simulink model "model_fallback"  (R2016a)
settings: Solver=VariableStepAuto  StartTime=0.0  StopTime=10.0  RelTol=1e-3
values from neighbouring files (symbols this model uses):
  alfa = 216.9    [init_fallback.m]
  g = 9.81    [init_fallback.m]
  L0 = 0.1255    [init_fallback.m]
  L1 = 0.05132    [init_fallback.m]
  m = 57.5    [init_fallback.m]
  R = 5.45    [init_fallback.m]
  x1zad = 0.015    [init_fallback.m]
undefined symbols (not defined in the file or in its folder): K, L
libraries: simulink x2
settings Model: Creator=Filip  LastModifiedBy=Filip

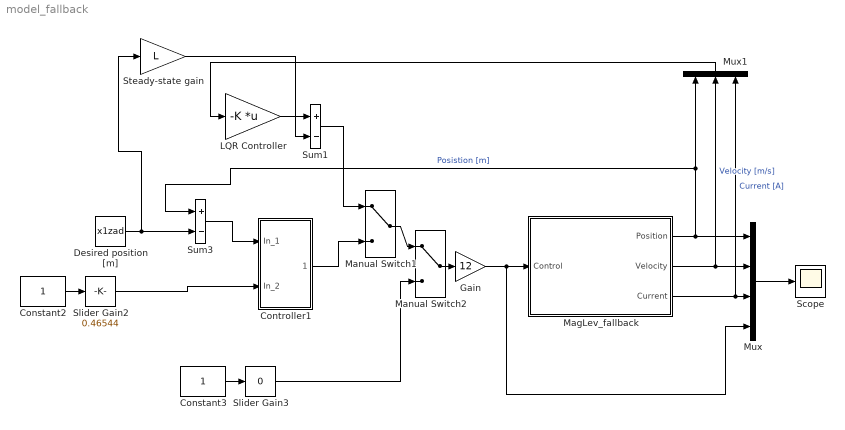
== system model_fallback ==
  Constant2 : Constant
  Constant3 : Constant
  Controller1 : Subsystem  mask(PID(2) Controller){P=40, I=3, D=0.5, T0=0.001}
      mask prompts: P "Proportional:"; I "Integral:"; D "Derivative:"; T0 "Sample Time:"
      mask help:
      | Enter Proportional(P), Integral(I), and Derivative(D) and divisor (N) terms.
      | P+I/s+Ds/(1/Ns+1)
      mask Help: This block implements a PID controller where parameters are entered for the Proportional, Integral and Derivative and divisor terms. Unmask this block to see how it works. The derivative term is implemented using an s/(s/N +1)  transfer function block. Making N large can create a "stiff" system.
      mask Display: disp('PID')
  "Desired position [m] " : Constant  Value=x1zad
  Gain : Gain  Gain=12
  LQR Controller : Gain  Gain=-K  Multiplication=Matrix(K*u)
  MagLev_fallback : Subsystem
  Manual Switch1 : ManualSwitch
  Manual Switch2 : ManualSwitch
  Mux : Mux
  Mux1 : Mux  Inputs=3
  Scope : Scope
  Slider Gain2 : simulink/Math Operations/Slider Gain  low=0  gain=0.46544  high=1
  Slider Gain3 : simulink/Math Operations/Slider Gain  low=0  gain=0  high=1
  Steady-state gain : Gain  Gain=L
  Sum1 : Sum  Inputs=+-  SaturateOnIntegerOverflow=on  InputSameDT=on  OutDataTypeStr=Inherit: Same as first input
  Sum3 : Sum  Inputs=+-  SaturateOnIntegerOverflow=on  InputSameDT=on  OutDataTypeStr=Inherit: Same as first input
  wires:
  Mux/1 -> Scope/1
  Gain/1 -> Mux/4, MagLev_fallback/1(Control)
  Manual Switch2/1 -> Gain/1
  MagLev_fallback/1(Position) -> Sum3/1, Mux1/1, Mux/1  "Posistion [m]"
  Constant2/1 -> Slider Gain2/1
  Slider Gain2/1 -> Controller1/2(In_2)
  "Desired position [m] "/1 -> Steady-state gain/1, Sum3/2
  Sum3/1 -> Controller1/1(In_1)
  Constant3/1 -> Slider Gain3/1
  Slider Gain3/1 -> Manual Switch2/2
  Manual Switch1/1 -> Manual Switch2/1
  Controller1/1(Out_1) -> Manual Switch1/2
  Mux1/1 -> LQR Controller/1
  LQR Controller/1 -> Sum1/1
  Sum1/1 -> Manual Switch1/1
  Steady-state gain/1 -> Sum1/2
  MagLev_fallback/2("Velocity ") -> Mux1/2, Mux/2  "Velocity [m/s]"
  MagLev_fallback/3(Current) -> Mux1/3, Mux/3  "Current [A]"

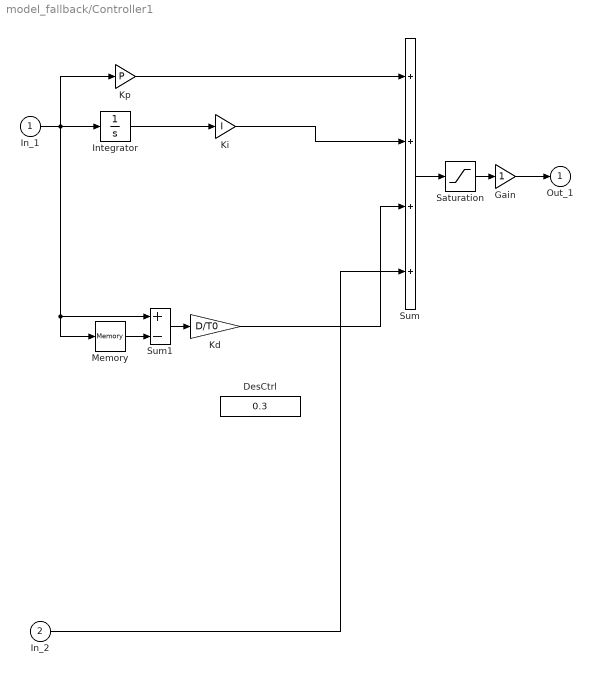
== system model_fallback/Controller1 ==
  In_1 : Inport
  In_2 : Inport  Port=2
  DesCtrl : Constant  Value=0.3
  Gain : Gain  SaturateOnIntegerOverflow=on  OutDataTypeStr=Inherit: Same as input  ParamDataTypeStr=Inherit: Same as input
  Integrator : Integrator  InitialCondition=0*4e-5  LimitOutput=on  UpperSaturationLimit=1  LowerSaturationLimit=-1
  Kd : Gain  Gain=D/T0  SaturateOnIntegerOverflow=on  OutDataTypeStr=Inherit: Same as input  ParamDataTypeStr=Inherit: Same as input
  Ki : Gain  Gain=I  SaturateOnIntegerOverflow=on  OutDataTypeStr=Inherit: Same as input  ParamDataTypeStr=Inherit: Same as input
  Kp : Gain  Gain=P  SaturateOnIntegerOverflow=on  OutDataTypeStr=Inherit: Same as input  ParamDataTypeStr=Inherit: Same as input
  Memory : Memory
  Saturation : Saturate  UpperLimit=1  LowerLimit=0
  Sum : Sum  Inputs=++++  SaturateOnIntegerOverflow=on  InputSameDT=on  OutDataTypeStr=Inherit: Same as first input
  Sum1 : Sum  Inputs=+-  SaturateOnIntegerOverflow=on  InputSameDT=on  OutDataTypeStr=Inherit: Same as first input
  Out_1 : Outport  InitialOutput=0
  wires:
  In_2/1 -> Sum/4
  Gain/1 -> Out_1/1
  Kd/1 -> Sum/3
  Kp/1 -> Sum/1
  Saturation/1 -> Gain/1
  Sum1/1 -> Kd/1
  Memory/1 -> Sum1/2
  In_1/1 -> Integrator/1, Sum1/1, Memory/1, Kp/1
  Sum/1 -> Saturation/1
  Integrator/1 -> Ki/1
  Ki/1 -> Sum/2

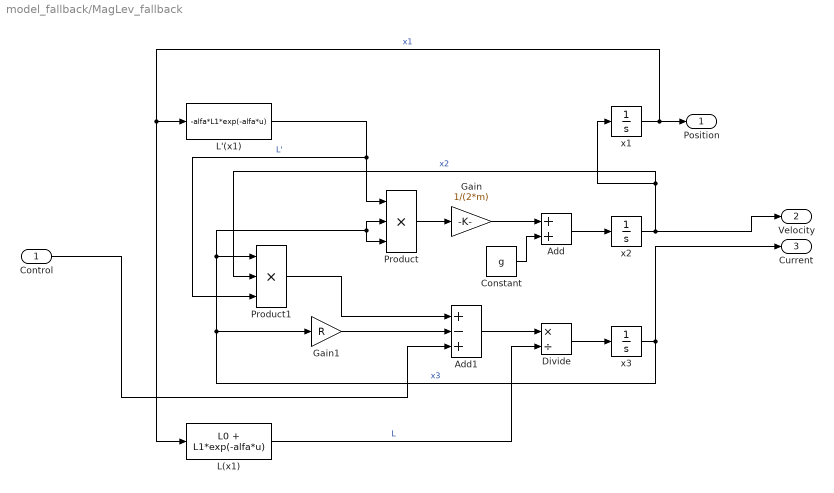
== system model_fallback/MagLev_fallback ==
  Control : Inport
  Add : Sum
  Add1 : Sum  Inputs=+-+
  Constant : Constant  Value=g
  Divide : Product  Inputs=*/
  Gain : Gain  Gain=1/(2*m)
  Gain1 : Gain  Gain=R
  L'(x1) : Fcn  Expr=-alfa*L1*exp(-alfa*u)
  L(x1) : Fcn  Expr=L0 + L1*exp(-alfa*u)
  Product : Product  Inputs=3
  Product1 : Product  Inputs=3
  x1 : Integrator
  x2 : Integrator
  x3 : Integrator
  Position : Outport
  "Velocity " : Outport  Port=2
  Current : Outport  Port=3
  wires:
  Gain/1 -> Add/1
  x2/1 -> "Velocity "/1, Product1/2, x1/1  "x2"
  Gain1/1 -> Add1/2
  Product1/1 -> Add1/1
  x1/1 -> L'(x1)/1, L(x1)/1, Position/1  "x1"
  L(x1)/1 -> Divide/2  "L"
  x3/1 -> Current/1, Product/3, Product/2, Product1/1, Gain1/1  "x3"
  Add/1 -> x2/1
  Constant/1 -> Add/2
  Product/1 -> Gain/1
  L'(x1)/1 -> Product1/3, Product/1  "L'"
  Divide/1 -> x3/1
  Add1/1 -> Divide/1
  Control/1 -> Add1/3
